simulink model "projektv3"  (R2025b)
settings: Solver=VariableStepAuto  StartTime=0.0  StopTime=2000  MaxStep=0.01  RelTol=1e-3
libraries: slpidlib x1
settings Model: Creator=admin  LastModifiedBy=roeberto
settings DataIOCC: ExternalInput=getinputstruct(spec1)  InitialState=getstatestruct(spec1)  LoadExternalInput=on  LoadInitialState=on
settings DebuggingCC: SignalInfNanChecking=error  IntegerSaturationMsg=error

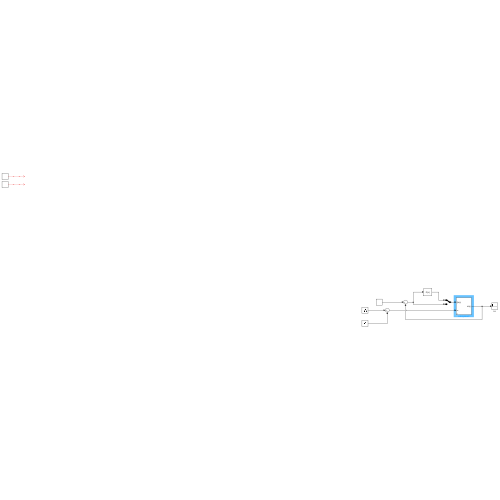
[thumbnail: Simulink's stored preview of the top-level diagram]
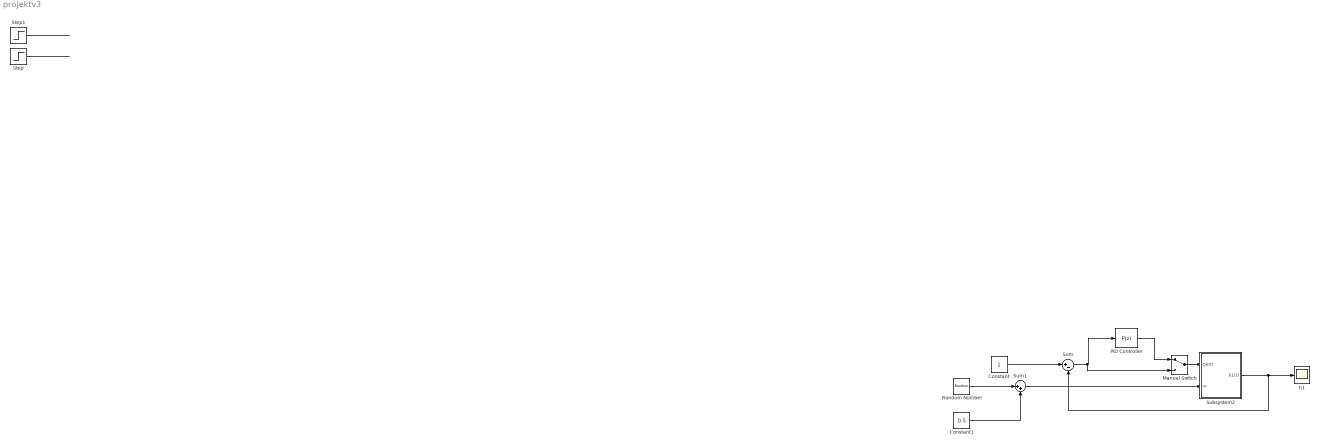
== system projektv3 ==
  Constant : Constant
  Constant1 : Constant  Value=0.5
  Manual Switch : ManualSwitch
  PID Controller : slpidlib/PID Controller  Controller=P  Form=Parallel  TimeDomain=Discrete-time  UseExternalTs=off  SampleTime=-1  IntegratorMethod=Forward Euler  FilterMethod=Forward Euler  ControllerParametersSource=internal  P=10  I=0.001  UseKiTs=off  D=1  UseExternalDerivativeSource=off  N=100  UseFilter=on  TunerSelectOption=Transfer Function Based (PID Tuner App)  InitialConditionSource=internal  InitialConditionForIntegrator=0  InitialConditionForFilter=0  DifferentiatorICPrevScaledInput=0  ExternalReset=none  TrackingMode=off  Kt=1  LimitOutput=off  SatLimitsSource=internal  UpperSaturationLimit=inf  LowerSaturationLimit=-inf  LinearizeAsGain=on  AntiWindupMode=none  Kb=1  LimitIntegrator=off  UpperIntegratorSaturationLimit=inf  LowerIntegratorSaturationLimit=-inf  POutMin=[]  POutMax=[]  IOutMin=[]  IOutMax=[]  DOutMin=[]  DOutMax=[]  NOutMin=[]  NOutMax=[]  SumOutMin=[]  SumOutMax=[]  SaturationOutMin=[]  SaturationOutMax=[]  PParamMin=[]  PParamMax=[]  IParamMin=[]  IParamMax=[]  DParamMin=[]  DParamMax=[]  NParamMin=[]  NParamMax=[]  KbParamMin=[]  KbParamMax=[]  KtParamMin=[]  KtParamMax=[]  KbOutMin=[]  KbOutMax=[]  KtOutMin=[]  KtOutMax=[]  IntegratorOutMin=[]  IntegratorOutMax=[]  FilterOutMin=[]  FilterOutMax=[]  SumI1OutMin=[]  SumI1OutMax=[]  SumI2OutMin=[]  SumI2OutMax=[]  SumI3OutMin=[]  SumI3OutMax=[]  SumI4OutMin=[]  SumI4OutMax=[]  SumDOutMin=[]  SumDOutMax=[]  DifferentiatorOutMin=[]  DifferentiatorOutMax=[]  FilterDiffOutCoefMin=[]  FilterDiffOutCoefMax=[]  ReciprocalOutMin=[]  ReciprocalOutMax=[]  SumDenOutMin=[]  SumDenOutMax=[]  SumNumOutMin=[]  SumNumOutMax=[]  DivideOutMin=[]  DivideOutMax=[]  UdiffTsProdOutMin=[]  UdiffTsProdOutMax=[]  NTsProdOutMin=[]  NTsProdOutMax=[]  UintegralTsProdOutMin=[]  UintegralTsProdOutMax=[]  UngainTsProdOutMin=[]  UngainTsProdOutMax=[]  ClampingZeroOutDataTypeStr=Inherit: Inherit via back propagation  ClampingZeroOutMin=[]  ClampingZeroOutMax=[]  FilterDenConstantOutDataTypeStr=Inherit: Inherit via back propagation  FilterDenConstantOutMin=[]  FilterDenConstantOutMax=[]  PCopyOutDataTypeStr=Inherit: Inherit via back propagation  PCopyOutMin=[]  PCopyOutMax=[]  NCopyOutDataTypeStr=Inherit: Inherit via back propagation  NCopyOutMin=[]  NCopyOutMax=[]  IntegratorContinuousStateAttributes=''  IntegratorStateMustResolveToSignalObject=off  IntegratorRTWStateStorageClass=Auto  FilterContinuousStateAttributes=''  FilterStateMustResolveToSignalObject=off  FilterRTWStateStorageClass=Auto  ParallelPVariant=InternalParameters  IdealPVariant=Disabled  IVariant=Disabled  DVariant=Disabled  IntegratorVariant=Disabled  SatVariant=Disabled  AWVariant=Disabled  PCopyVariant=Disabled  TRVariant=Disabled  FdbkBlocksVariant=Forward  IdealPFdbkVariant=Disabled  SatFdbkVariant=Disabled  DerivativeFilterVariant=Disabled  NVariant=Disabled  NCopyVariant=Disabled_SignalSpec  FilterICVariant=Disabled  IntegratorICVariant=Disabled  ExternalResetVariant=Disabled  TRSumVariant=Passthrough  SumFdbkVariant=Disabled  SumVariant=Passthrough_P  TsampFilterVariant=InternalTs  TsampNgainVariant=Passthrough  TsampIntegralVariant=Disabled_SignalSpec  ExternalSaturationOutDataTypeStr=Inherit: Same as second input  DerivativeSourceVariant=Disabled  PreIntVariant=InternalPreInt
  Random Number : RandomNumber  Mean=5  Variance=100  Seed=87453  SampleTime=10
  Step : Step  Time=0  After=0.01  SampleTime=0
  Step1 : Step  Time=0  After=0.01  SampleTime=0
  Subsystem2 : Subsystem  mask{h10=2, h20=0.001, r1=1, r2=1, H1=2, H2=2, rr=0.05, rv=0.04, g=9.81, m1=300, m2=300, ur=0.95}
      mask prompts: r1 "promień podstawy zbiornika 1"; r2 "promień podstawy zbiornika 2"; H1 "Wysokość zbiornika 1"; H2 "Wysokość zbiornika 2"; rr "promień kryzy"; rv "promień kryzy"; g "przyspieszenie grawitacyjne"; m1 "masa zbiornika 1"; m2 "masa zbiornika 2"; ur "współczynnik wypływu kryzy"
      mask DialogControl Container3 Prompt: Warunki początkowe
      mask DialogControl ParameterGroupVar Prompt: Parametry modelu
  Sum : Sum  Inputs=|+-
  Sum1 : Sum  Inputs=|++
  h1 : Scope
      settings: ActiveDisplayYMinimum=-0.080893622135050025  ActiveDisplayYMaximum=2.4821224039953531
  wires:
  Step1/1 -> ?
  Step/1 -> ?
  Constant/1 -> Sum/1
  Subsystem2/1(h1(t)) -> h1/1, Sum/2
  Random Number/1 -> Sum1/1
  Sum1/1 -> Subsystem2/2(ur)
  Constant1/1 -> Sum1/2
  Sum/1 -> Manual Switch/2, PID Controller/1
  Manual Switch/1 -> Subsystem2/1(Qh(t))
  PID Controller/1 -> Manual Switch/1

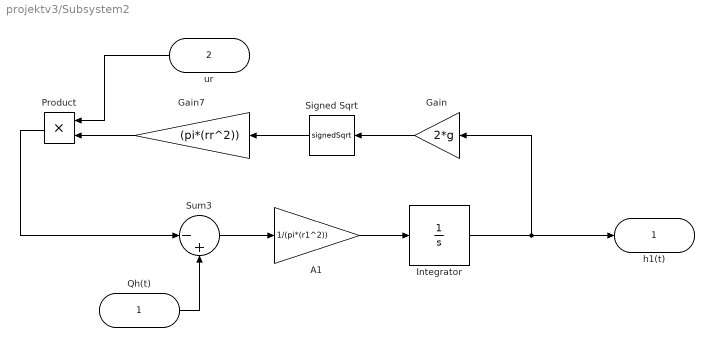
== system projektv3/Subsystem2 ==
  Qh(t) : Inport
  ur : Inport  Port=2
  A1 : Gain  Gain=1/(pi*(r1^2))
  Gain : Gain  Gain=2*g
  Gain7 : Gain  Gain=(pi*(rr^2))
  Integrator : Integrator  InitialCondition=h10  LimitOutput=on  UpperSaturationLimit=H1  LowerSaturationLimit=0.001
  Product : Product
  Signed Sqrt : Sqrt  Operator=signedSqrt
  Sum3 : Sum  Inputs=|-+
  h1(t) : Outport  OutMin=0.001  OutMax=H1
  wires:
  A1/1 -> Integrator/1
  Signed Sqrt/1 -> Gain7/1
  Sum3/1 -> A1/1
  Integrator/1 -> Gain/1, h1(t)/1
  Gain/1 -> Signed Sqrt/1
  Qh(t)/1 -> Sum3/2
  ur/1 -> Product/1
  Gain7/1 -> Product/2
  Product/1 -> Sum3/1
